simulink model "VDCHyd2020a"  (R2020a)
settings: Solver=daessc  StartTime=0.0  StopTime=simulationEndTime  FixedStep=0.001  RelTol=1e-2
values from neighbouring files (symbols this model uses):
  Bc1_V = [0;0;0;0;0;0]    [initializeSimulationGP.m]
  filtDV = init2ndOrderLowPassFilter(35*2*pi,1,controller.dT)    [initializeLowPassFilters.m]
  filtEnc = init2ndOrderLowPassFilter(35*2*pi,1,controller.dT)    [initializeLowPassFilters.m]
undefined symbols (not defined in the file or in its folder): aux, B11_r_B11Tc1, B11_V, B11_Vr, B11Ftot_r, B12_r_B12Tc2, B12_Rot_Tc2, B12_U_Tc2, B12_V, B12_Vr, B12Ftot_r, B31_r_B31B41, B31_V, B31_Vr, B31FTot_r, B32_r_B32B42, B32_Rot_B42, B32_U_B42, B32_V, B32_Vr, B32FTot_r, B41_r_B41Tc1, B41_V, B41_Vr, B41FTot_r, B42_r_B42Tc2, B42_Rot_Tc2, B42_U_Tc2, B42_V, B42_Vr, B42FTot_r, B52_r_B52P32, B52_Rot_P32, B52_U_P32, B52_V, B52_Vr, B52Ftot_r, Bc1_r_Bc1B11, Bc1_r_Bc1B31, Bc1_Vr, Bc1FTot_r, Bc2_r_Bc2B12, Bc2_r_Bc2B32, Bc2_Rot_B12, Bc2_Rot_B32, Bc2_U_B12, Bc2_U_B32, Bc2_V, Bc2_Vr, Bc2Tot_r, controller, cyl1, cyl2, cylT2, D22_V, D22_Vr, D22Fr, DiscIntNeverNeededParam, dq1, dq11 ... (+125)
libraries: sm_lib x34, nesl_utility x15, simulink x11, dspinverses x1
(part 10 of 12)

== system VDCHyd2020a/sbVDCController/sbFormTotalRequiredForces/sbTotalRequiredForcesRS2/sbFilteredVelocityDerivativeB42/sbDiscreteDerivative3 ==
  u : Inport
  Add : Sum  Inputs=-+
  Gain6 : Gain  Gain=1/(2*controller.dT)
  Integer Delay : Delay  InitialConditionSource=Input port  InitialCondition=0  SampleTime=controller.dT
      settings: InputPortMap=u0,p4
  du/dt : Outport  PortDimensions=1
  wires:
  Add/1 -> Gain6/1
  Integer Delay/1 -> Add/1
  u/1 -> Integer Delay/1, Integer Delay/2, Add/2
  Gain6/1 -> du/dt/1

== system VDCHyd2020a/sbVDCController/sbFormTotalRequiredForces/sbTotalRequiredForcesRS2/sbFilteredVelocityDerivativeB42/sbDiscreteDerivative4 ==
  u : Inport
  Add : Sum  Inputs=-+
  Gain6 : Gain  Gain=1/(2*controller.dT)
  Integer Delay : Delay  InitialConditionSource=Input port  InitialCondition=0  SampleTime=controller.dT
      settings: InputPortMap=u0,p4
  du/dt : Outport  PortDimensions=1
  wires:
  Add/1 -> Gain6/1
  Integer Delay/1 -> Add/1
  u/1 -> Integer Delay/1, Integer Delay/2, Add/2
  Gain6/1 -> du/dt/1

== system VDCHyd2020a/sbVDCController/sbFormTotalRequiredForces/sbTotalRequiredForcesRS2/sbFilteredVelocityDerivativeB42/sbDiscreteDerivative5 ==
  u : Inport
  Add : Sum  Inputs=-+
  Gain6 : Gain  Gain=1/(2*controller.dT)
  Integer Delay : Delay  InitialConditionSource=Input port  InitialCondition=0  SampleTime=controller.dT
      settings: InputPortMap=u0,p4
  du/dt : Outport  PortDimensions=1
  wires:
  Add/1 -> Gain6/1
  Integer Delay/1 -> Add/1
  u/1 -> Integer Delay/1, Integer Delay/2, Add/2
  Gain6/1 -> du/dt/1

== system VDCHyd2020a/sbVDCController/sbFormTotalRequiredForces/sbTotalRequiredForcesRS2/sbFilteredVelocityDerivativeB42/sbDiscreteDerivative6 ==
  u : Inport
  Add : Sum  Inputs=-+
  Gain6 : Gain  Gain=1/(2*controller.dT)
  Integer Delay : Delay  InitialConditionSource=Input port  InitialCondition=0  SampleTime=controller.dT
      settings: InputPortMap=u0,p4
  du/dt : Outport  PortDimensions=1
  wires:
  Add/1 -> Gain6/1
  Integer Delay/1 -> Add/1
  u/1 -> Integer Delay/1, Integer Delay/2, Add/2
  Gain6/1 -> du/dt/1

== system VDCHyd2020a/sbVDCController/sbFormTotalRequiredForces/sbTotalRequiredForcesRS2/sbFilteredVelocityDerivativeB42/sbLowPassFilter1 ==
  dV : Inport
  Delay : Delay  InitialConditionSource=Input port  SampleTime=filtDV.dT
      settings: InputPortMap=u0,p4
  Delay1 : Delay  DelayLength=1  InitialConditionSource=Input port  SampleTime=filtDV.dT
      settings: InputPortMap=u0,p4
  Delay2 : Delay  DelayLength=0  InitialConditionSource=Input port  SampleTime=filtDV.dT
      settings: InputPortMap=u0,p4
  Delay3 : Delay  InitialConditionSource=Input port  SampleTime=filtDV.dT
      settings: InputPortMap=u0,p4
  Delay4 : Delay  DelayLength=1  InitialConditionSource=Input port  SampleTime=filtDV.dT
      settings: InputPortMap=u0,p4
  Gain : Gain  Gain=filtDV.a0
  Gain1 : Gain  Gain=filtDV.b1
  Gain2 : Gain  Gain=filtDV.b2
  Gain3 : Gain  Gain=filtDV.b0
  Gain4 : Gain  Gain=filtDV.a1
  Sum : Sum  Inputs=|--+++
  dVFilt : Outport
  wires:
  Gain3/1 -> Sum/5
  Gain2/1 -> Sum/3
  Delay4/1 -> Gain4/1
  Delay/1 -> Gain/1
  Delay1/1 -> Gain1/1
  Delay2/1 -> Gain2/1
  Gain4/1 -> Sum/1
  Sum/1 -> dVFilt/1, Delay4/1, Delay/1  "dVFilt"
  dV/1 -> Delay2/1, Delay2/2, Delay1/1, Delay3/2, Delay3/1, Delay1/2, Delay4/2, Delay/2  "dV"
  Gain1/1 -> Sum/4
  Gain/1 -> Sum/2
  Delay3/1 -> Gain3/1

== system VDCHyd2020a/sbVDCController/sbFormTotalRequiredForces/sbTotalRequiredForcesRS2/sbFilteredVelocityDerivativeB42/sbLowPassFilter2 ==
  dV : Inport
  Delay : Delay  InitialConditionSource=Input port  SampleTime=filtDV.dT
      settings: InputPortMap=u0,p4
  Delay1 : Delay  DelayLength=1  InitialConditionSource=Input port  SampleTime=filtDV.dT
      settings: InputPortMap=u0,p4
  Delay2 : Delay  DelayLength=0  InitialConditionSource=Input port  SampleTime=filtDV.dT
      settings: InputPortMap=u0,p4
  Delay3 : Delay  InitialConditionSource=Input port  SampleTime=filtDV.dT
      settings: InputPortMap=u0,p4
  Delay4 : Delay  DelayLength=1  InitialConditionSource=Input port  SampleTime=filtDV.dT
      settings: InputPortMap=u0,p4
  Gain : Gain  Gain=filtDV.a0
  Gain1 : Gain  Gain=filtDV.b1
  Gain2 : Gain  Gain=filtDV.b2
  Gain3 : Gain  Gain=filtDV.b0
  Gain4 : Gain  Gain=filtDV.a1
  Sum : Sum  Inputs=|--+++
  dVFilt : Outport
  wires:
  Delay3/1 -> Gain3/1
  Gain/1 -> Sum/2
  Gain1/1 -> Sum/4
  dV/1 -> Delay/2, Delay4/2, Delay1/2, Delay3/1, Delay3/2, Delay1/1, Delay2/2, Delay2/1  "dV"
  Sum/1 -> Delay/1, Delay4/1, dVFilt/1  "dVFilt"
  Gain4/1 -> Sum/1
  Delay2/1 -> Gain2/1
  Delay1/1 -> Gain1/1
  Delay/1 -> Gain/1
  Delay4/1 -> Gain4/1
  Gain2/1 -> Sum/3
  Gain3/1 -> Sum/5

== system VDCHyd2020a/sbVDCController/sbFormTotalRequiredForces/sbTotalRequiredForcesRS2/sbFilteredVelocityDerivativeB42/sbLowPassFilter3 ==
  dV : Inport
  Delay : Delay  InitialConditionSource=Input port  SampleTime=filtDV.dT
      settings: InputPortMap=u0,p4
  Delay1 : Delay  DelayLength=1  InitialConditionSource=Input port  SampleTime=filtDV.dT
      settings: InputPortMap=u0,p4
  Delay2 : Delay  DelayLength=0  InitialConditionSource=Input port  SampleTime=filtDV.dT
      settings: InputPortMap=u0,p4
  Delay3 : Delay  InitialConditionSource=Input port  SampleTime=filtDV.dT
      settings: InputPortMap=u0,p4
  Delay4 : Delay  DelayLength=1  InitialConditionSource=Input port  SampleTime=filtDV.dT
      settings: InputPortMap=u0,p4
  Gain : Gain  Gain=filtDV.a0
  Gain1 : Gain  Gain=filtDV.b1
  Gain2 : Gain  Gain=filtDV.b2
  Gain3 : Gain  Gain=filtDV.b0
  Gain4 : Gain  Gain=filtDV.a1
  Sum : Sum  Inputs=|--+++
  dVFilt : Outport
  wires:
  Gain3/1 -> Sum/5
  Gain2/1 -> Sum/3
  Delay4/1 -> Gain4/1
  Delay/1 -> Gain/1
  Delay1/1 -> Gain1/1
  Delay2/1 -> Gain2/1
  Gain4/1 -> Sum/1
  Sum/1 -> dVFilt/1, Delay4/1, Delay/1  "dVFilt"
  dV/1 -> Delay2/1, Delay2/2, Delay1/1, Delay3/2, Delay3/1, Delay1/2, Delay4/2, Delay/2  "dV"
  Gain1/1 -> Sum/4
  Gain/1 -> Sum/2
  Delay3/1 -> Gain3/1

== system VDCHyd2020a/sbVDCController/sbFormTotalRequiredForces/sbTotalRequiredForcesRS2/sbFilteredVelocityDerivativeB42/sbLowPassFilter4 ==
  dV : Inport
  Delay : Delay  InitialConditionSource=Input port  SampleTime=filtDV.dT
      settings: InputPortMap=u0,p4
  Delay1 : Delay  DelayLength=1  InitialConditionSource=Input port  SampleTime=filtDV.dT
      settings: InputPortMap=u0,p4
  Delay2 : Delay  DelayLength=0  InitialConditionSource=Input port  SampleTime=filtDV.dT
      settings: InputPortMap=u0,p4
  Delay3 : Delay  InitialConditionSource=Input port  SampleTime=filtDV.dT
      settings: InputPortMap=u0,p4
  Delay4 : Delay  DelayLength=1  InitialConditionSource=Input port  SampleTime=filtDV.dT
      settings: InputPortMap=u0,p4
  Gain : Gain  Gain=filtDV.a0
  Gain1 : Gain  Gain=filtDV.b1
  Gain2 : Gain  Gain=filtDV.b2
  Gain3 : Gain  Gain=filtDV.b0
  Gain4 : Gain  Gain=filtDV.a1
  Sum : Sum  Inputs=|--+++
  dVFilt : Outport
  wires:
  Delay3/1 -> Gain3/1
  Gain/1 -> Sum/2
  Gain1/1 -> Sum/4
  dV/1 -> Delay/2, Delay4/2, Delay1/2, Delay3/1, Delay3/2, Delay1/1, Delay2/2, Delay2/1  "dV"
  Sum/1 -> Delay/1, Delay4/1, dVFilt/1  "dVFilt"
  Gain4/1 -> Sum/1
  Delay2/1 -> Gain2/1
  Delay1/1 -> Gain1/1
  Delay/1 -> Gain/1
  Delay4/1 -> Gain4/1
  Gain2/1 -> Sum/3
  Gain3/1 -> Sum/5

== system VDCHyd2020a/sbVDCController/sbFormTotalRequiredForces/sbTotalRequiredForcesRS2/sbFilteredVelocityDerivativeB42/sbLowPassFilter5 ==
  dV : Inport
  Delay : Delay  InitialConditionSource=Input port  SampleTime=filtDV.dT
      settings: InputPortMap=u0,p4
  Delay1 : Delay  DelayLength=1  InitialConditionSource=Input port  SampleTime=filtDV.dT
      settings: InputPortMap=u0,p4
  Delay2 : Delay  DelayLength=0  InitialConditionSource=Input port  SampleTime=filtDV.dT
      settings: InputPortMap=u0,p4
  Delay3 : Delay  InitialConditionSource=Input port  SampleTime=filtDV.dT
      settings: InputPortMap=u0,p4
  Delay4 : Delay  DelayLength=1  InitialConditionSource=Input port  SampleTime=filtDV.dT
      settings: InputPortMap=u0,p4
  Gain : Gain  Gain=filtDV.a0
  Gain1 : Gain  Gain=filtDV.b1
  Gain2 : Gain  Gain=filtDV.b2
  Gain3 : Gain  Gain=filtDV.b0
  Gain4 : Gain  Gain=filtDV.a1
  Sum : Sum  Inputs=|--+++
  dVFilt : Outport
  wires:
  Gain3/1 -> Sum/5
  Gain2/1 -> Sum/3
  Delay4/1 -> Gain4/1
  Delay/1 -> Gain/1
  Delay1/1 -> Gain1/1
  Delay2/1 -> Gain2/1
  Gain4/1 -> Sum/1
  Sum/1 -> dVFilt/1, Delay4/1, Delay/1  "dVFilt"
  dV/1 -> Delay2/1, Delay2/2, Delay1/1, Delay3/2, Delay3/1, Delay1/2, Delay4/2, Delay/2  "dV"
  Gain1/1 -> Sum/4
  Gain/1 -> Sum/2
  Delay3/1 -> Gain3/1

== system VDCHyd2020a/sbVDCController/sbFormTotalRequiredForces/sbTotalRequiredForcesRS2/sbFilteredVelocityDerivativeB42/sbLowPassFilter6 ==
  dV : Inport
  Delay : Delay  InitialConditionSource=Input port  SampleTime=filtDV.dT
      settings: InputPortMap=u0,p4
  Delay1 : Delay  DelayLength=1  InitialConditionSource=Input port  SampleTime=filtDV.dT
      settings: InputPortMap=u0,p4
  Delay2 : Delay  DelayLength=0  InitialConditionSource=Input port  SampleTime=filtDV.dT
      settings: InputPortMap=u0,p4
  Delay3 : Delay  InitialConditionSource=Input port  SampleTime=filtDV.dT
      settings: InputPortMap=u0,p4
  Delay4 : Delay  DelayLength=1  InitialConditionSource=Input port  SampleTime=filtDV.dT
      settings: InputPortMap=u0,p4
  Gain : Gain  Gain=filtDV.a0
  Gain1 : Gain  Gain=filtDV.b1
  Gain2 : Gain  Gain=filtDV.b2
  Gain3 : Gain  Gain=filtDV.b0
  Gain4 : Gain  Gain=filtDV.a1
  Sum : Sum  Inputs=|--+++
  dVFilt : Outport
  wires:
  Delay3/1 -> Gain3/1
  Gain/1 -> Sum/2
  Gain1/1 -> Sum/4
  dV/1 -> Delay/2, Delay4/2, Delay1/2, Delay3/1, Delay3/2, Delay1/1, Delay2/2, Delay2/1  "dV"
  Sum/1 -> Delay/1, Delay4/1, dVFilt/1  "dVFilt"
  Gain4/1 -> Sum/1
  Delay2/1 -> Gain2/1
  Delay1/1 -> Gain1/1
  Delay/1 -> Gain/1
  Delay4/1 -> Gain4/1
  Gain2/1 -> Sum/3
  Gain3/1 -> Sum/5

== system VDCHyd2020a/sbVDCController/sbFormTotalRequiredForces/sbTotalRequiredForcesRS2/sbFilteredVelocityDerivativeBc2/sbDiscreteDerivative1 ==
  u : Inport
  Add : Sum  Inputs=-+
  Gain6 : Gain  Gain=1/(2*controller.dT)
  Integer Delay : Delay  InitialConditionSource=Input port  InitialCondition=0  SampleTime=controller.dT
      settings: InputPortMap=u0,p4
  du/dt : Outport  PortDimensions=1
  wires:
  Add/1 -> Gain6/1
  u/1 -> Integer Delay/1, Integer Delay/2, Add/2
  Integer Delay/1 -> Add/1
  Gain6/1 -> du/dt/1

== system VDCHyd2020a/sbVDCController/sbFormTotalRequiredForces/sbTotalRequiredForcesRS2/sbFilteredVelocityDerivativeBc2/sbDiscreteDerivative2 ==
  u : Inport
  Add : Sum  Inputs=-+
  Gain6 : Gain  Gain=1/(2*controller.dT)
  Integer Delay : Delay  InitialConditionSource=Input port  InitialCondition=0  SampleTime=controller.dT
      settings: InputPortMap=u0,p4
  du/dt : Outport  PortDimensions=1
  wires:
  u/1 -> Integer Delay/1, Integer Delay/2, Add/2
  Integer Delay/1 -> Add/1
  Add/1 -> Gain6/1
  Gain6/1 -> du/dt/1

== system VDCHyd2020a/sbVDCController/sbFormTotalRequiredForces/sbTotalRequiredForcesRS2/sbFilteredVelocityDerivativeBc2/sbDiscreteDerivative3 ==
  u : Inport
  Add : Sum  Inputs=-+
  Gain6 : Gain  Gain=1/(2*controller.dT)
  Integer Delay : Delay  InitialConditionSource=Input port  InitialCondition=0  SampleTime=controller.dT
      settings: InputPortMap=u0,p4
  du/dt : Outport  PortDimensions=1
  wires:
  Add/1 -> Gain6/1
  Integer Delay/1 -> Add/1
  u/1 -> Integer Delay/1, Integer Delay/2, Add/2
  Gain6/1 -> du/dt/1

== system VDCHyd2020a/sbVDCController/sbFormTotalRequiredForces/sbTotalRequiredForcesRS2/sbFilteredVelocityDerivativeBc2/sbDiscreteDerivative4 ==
  u : Inport
  Add : Sum  Inputs=-+
  Gain6 : Gain  Gain=1/(2*controller.dT)
  Integer Delay : Delay  InitialConditionSource=Input port  InitialCondition=0  SampleTime=controller.dT
      settings: InputPortMap=u0,p4
  du/dt : Outport  PortDimensions=1
  wires:
  Add/1 -> Gain6/1
  Integer Delay/1 -> Add/1
  u/1 -> Integer Delay/1, Integer Delay/2, Add/2
  Gain6/1 -> du/dt/1

== system VDCHyd2020a/sbVDCController/sbFormTotalRequiredForces/sbTotalRequiredForcesRS2/sbFilteredVelocityDerivativeBc2/sbDiscreteDerivative5 ==
  u : Inport
  Add : Sum  Inputs=-+
  Gain6 : Gain  Gain=1/(2*controller.dT)
  Integer Delay : Delay  InitialConditionSource=Input port  InitialCondition=0  SampleTime=controller.dT
      settings: InputPortMap=u0,p4
  du/dt : Outport  PortDimensions=1
  wires:
  Add/1 -> Gain6/1
  Integer Delay/1 -> Add/1
  u/1 -> Integer Delay/1, Integer Delay/2, Add/2
  Gain6/1 -> du/dt/1

== system VDCHyd2020a/sbVDCController/sbFormTotalRequiredForces/sbTotalRequiredForcesRS2/sbFilteredVelocityDerivativeBc2/sbDiscreteDerivative6 ==
  u : Inport
  Add : Sum  Inputs=-+
  Gain6 : Gain  Gain=1/(2*controller.dT)
  Integer Delay : Delay  InitialConditionSource=Input port  InitialCondition=0  SampleTime=controller.dT
      settings: InputPortMap=u0,p4
  du/dt : Outport  PortDimensions=1
  wires:
  Add/1 -> Gain6/1
  Integer Delay/1 -> Add/1
  u/1 -> Integer Delay/1, Integer Delay/2, Add/2
  Gain6/1 -> du/dt/1

== system VDCHyd2020a/sbVDCController/sbFormTotalRequiredForces/sbTotalRequiredForcesRS2/sbFilteredVelocityDerivativeBc2/sbLowPassFilter1 ==
  dV : Inport
  Delay : Delay  InitialConditionSource=Input port  SampleTime=filtDV.dT
      settings: InputPortMap=u0,p4
  Delay1 : Delay  DelayLength=1  InitialConditionSource=Input port  SampleTime=filtDV.dT
      settings: InputPortMap=u0,p4
  Delay2 : Delay  DelayLength=0  InitialConditionSource=Input port  SampleTime=filtDV.dT
      settings: InputPortMap=u0,p4
  Delay3 : Delay  InitialConditionSource=Input port  SampleTime=filtDV.dT
      settings: InputPortMap=u0,p4
  Delay4 : Delay  DelayLength=1  InitialConditionSource=Input port  SampleTime=filtDV.dT
      settings: InputPortMap=u0,p4
  Gain : Gain  Gain=filtDV.a0
  Gain1 : Gain  Gain=filtDV.b1
  Gain2 : Gain  Gain=filtDV.b2
  Gain3 : Gain  Gain=filtDV.b0
  Gain4 : Gain  Gain=filtDV.a1
  Sum : Sum  Inputs=|--+++
  dVFilt : Outport
  wires:
  Gain3/1 -> Sum/5
  Gain2/1 -> Sum/3
  Delay4/1 -> Gain4/1
  Delay/1 -> Gain/1
  Delay1/1 -> Gain1/1
  Delay2/1 -> Gain2/1
  Gain4/1 -> Sum/1
  Sum/1 -> dVFilt/1, Delay4/1, Delay/1  "dVFilt"
  dV/1 -> Delay2/1, Delay2/2, Delay1/1, Delay3/2, Delay3/1, Delay1/2, Delay4/2, Delay/2  "dV"
  Gain1/1 -> Sum/4
  Gain/1 -> Sum/2
  Delay3/1 -> Gain3/1

== system VDCHyd2020a/sbVDCController/sbFormTotalRequiredForces/sbTotalRequiredForcesRS2/sbFilteredVelocityDerivativeBc2/sbLowPassFilter2 ==
  dV : Inport
  Delay : Delay  InitialConditionSource=Input port  SampleTime=filtDV.dT
      settings: InputPortMap=u0,p4
  Delay1 : Delay  DelayLength=1  InitialConditionSource=Input port  SampleTime=filtDV.dT
      settings: InputPortMap=u0,p4
  Delay2 : Delay  DelayLength=0  InitialConditionSource=Input port  SampleTime=filtDV.dT
      settings: InputPortMap=u0,p4
  Delay3 : Delay  InitialConditionSource=Input port  SampleTime=filtDV.dT
      settings: InputPortMap=u0,p4
  Delay4 : Delay  DelayLength=1  InitialConditionSource=Input port  SampleTime=filtDV.dT
      settings: InputPortMap=u0,p4
  Gain : Gain  Gain=filtDV.a0
  Gain1 : Gain  Gain=filtDV.b1
  Gain2 : Gain  Gain=filtDV.b2
  Gain3 : Gain  Gain=filtDV.b0
  Gain4 : Gain  Gain=filtDV.a1
  Sum : Sum  Inputs=|--+++
  dVFilt : Outport
  wires:
  Delay3/1 -> Gain3/1
  Gain/1 -> Sum/2
  Gain1/1 -> Sum/4
  dV/1 -> Delay/2, Delay4/2, Delay1/2, Delay3/1, Delay3/2, Delay1/1, Delay2/2, Delay2/1  "dV"
  Sum/1 -> Delay/1, Delay4/1, dVFilt/1  "dVFilt"
  Gain4/1 -> Sum/1
  Delay2/1 -> Gain2/1
  Delay1/1 -> Gain1/1
  Delay/1 -> Gain/1
  Delay4/1 -> Gain4/1
  Gain2/1 -> Sum/3
  Gain3/1 -> Sum/5

== system VDCHyd2020a/sbVDCController/sbFormTotalRequiredForces/sbTotalRequiredForcesRS2/sbFilteredVelocityDerivativeBc2/sbLowPassFilter3 ==
  dV : Inport
  Delay : Delay  InitialConditionSource=Input port  SampleTime=filtDV.dT
      settings: InputPortMap=u0,p4
  Delay1 : Delay  DelayLength=1  InitialConditionSource=Input port  SampleTime=filtDV.dT
      settings: InputPortMap=u0,p4
  Delay2 : Delay  DelayLength=0  InitialConditionSource=Input port  SampleTime=filtDV.dT
      settings: InputPortMap=u0,p4
  Delay3 : Delay  InitialConditionSource=Input port  SampleTime=filtDV.dT
      settings: InputPortMap=u0,p4
  Delay4 : Delay  DelayLength=1  InitialConditionSource=Input port  SampleTime=filtDV.dT
      settings: InputPortMap=u0,p4
  Gain : Gain  Gain=filtDV.a0
  Gain1 : Gain  Gain=filtDV.b1
  Gain2 : Gain  Gain=filtDV.b2
  Gain3 : Gain  Gain=filtDV.b0
  Gain4 : Gain  Gain=filtDV.a1
  Sum : Sum  Inputs=|--+++
  dVFilt : Outport
  wires:
  Gain3/1 -> Sum/5
  Gain2/1 -> Sum/3
  Delay4/1 -> Gain4/1
  Delay/1 -> Gain/1
  Delay1/1 -> Gain1/1
  Delay2/1 -> Gain2/1
  Gain4/1 -> Sum/1
  Sum/1 -> dVFilt/1, Delay4/1, Delay/1  "dVFilt"
  dV/1 -> Delay2/1, Delay2/2, Delay1/1, Delay3/2, Delay3/1, Delay1/2, Delay4/2, Delay/2  "dV"
  Gain1/1 -> Sum/4
  Gain/1 -> Sum/2
  Delay3/1 -> Gain3/1

== system VDCHyd2020a/sbVDCController/sbFormTotalRequiredForces/sbTotalRequiredForcesRS2/sbFilteredVelocityDerivativeBc2/sbLowPassFilter4 ==
  dV : Inport
  Delay : Delay  InitialConditionSource=Input port  SampleTime=filtDV.dT
      settings: InputPortMap=u0,p4
  Delay1 : Delay  DelayLength=1  InitialConditionSource=Input port  SampleTime=filtDV.dT
      settings: InputPortMap=u0,p4
  Delay2 : Delay  DelayLength=0  InitialConditionSource=Input port  SampleTime=filtDV.dT
      settings: InputPortMap=u0,p4
  Delay3 : Delay  InitialConditionSource=Input port  SampleTime=filtDV.dT
      settings: InputPortMap=u0,p4
  Delay4 : Delay  DelayLength=1  InitialConditionSource=Input port  SampleTime=filtDV.dT
      settings: InputPortMap=u0,p4
  Gain : Gain  Gain=filtDV.a0
  Gain1 : Gain  Gain=filtDV.b1
  Gain2 : Gain  Gain=filtDV.b2
  Gain3 : Gain  Gain=filtDV.b0
  Gain4 : Gain  Gain=filtDV.a1
  Sum : Sum  Inputs=|--+++
  dVFilt : Outport
  wires:
  Delay3/1 -> Gain3/1
  Gain/1 -> Sum/2
  Gain1/1 -> Sum/4
  dV/1 -> Delay/2, Delay4/2, Delay1/2, Delay3/1, Delay3/2, Delay1/1, Delay2/2, Delay2/1  "dV"
  Sum/1 -> Delay/1, Delay4/1, dVFilt/1  "dVFilt"
  Gain4/1 -> Sum/1
  Delay2/1 -> Gain2/1
  Delay1/1 -> Gain1/1
  Delay/1 -> Gain/1
  Delay4/1 -> Gain4/1
  Gain2/1 -> Sum/3
  Gain3/1 -> Sum/5

== system VDCHyd2020a/sbVDCController/sbFormTotalRequiredForces/sbTotalRequiredForcesRS2/sbFilteredVelocityDerivativeBc2/sbLowPassFilter5 ==
  dV : Inport
  Delay : Delay  InitialConditionSource=Input port  SampleTime=filtDV.dT
      settings: InputPortMap=u0,p4
  Delay1 : Delay  DelayLength=1  InitialConditionSource=Input port  SampleTime=filtDV.dT
      settings: InputPortMap=u0,p4
  Delay2 : Delay  DelayLength=0  InitialConditionSource=Input port  SampleTime=filtDV.dT
      settings: InputPortMap=u0,p4
  Delay3 : Delay  InitialConditionSource=Input port  SampleTime=filtDV.dT
      settings: InputPortMap=u0,p4
  Delay4 : Delay  DelayLength=1  InitialConditionSource=Input port  SampleTime=filtDV.dT
      settings: InputPortMap=u0,p4
  Gain : Gain  Gain=filtDV.a0
  Gain1 : Gain  Gain=filtDV.b1
  Gain2 : Gain  Gain=filtDV.b2
  Gain3 : Gain  Gain=filtDV.b0
  Gain4 : Gain  Gain=filtDV.a1
  Sum : Sum  Inputs=|--+++
  dVFilt : Outport
  wires:
  Gain3/1 -> Sum/5
  Gain2/1 -> Sum/3
  Delay4/1 -> Gain4/1
  Delay/1 -> Gain/1
  Delay1/1 -> Gain1/1
  Delay2/1 -> Gain2/1
  Gain4/1 -> Sum/1
  Sum/1 -> dVFilt/1, Delay4/1, Delay/1  "dVFilt"
  dV/1 -> Delay2/1, Delay2/2, Delay1/1, Delay3/2, Delay3/1, Delay1/2, Delay4/2, Delay/2  "dV"
  Gain1/1 -> Sum/4
  Gain/1 -> Sum/2
  Delay3/1 -> Gain3/1

== system VDCHyd2020a/sbVDCController/sbFormTotalRequiredForces/sbTotalRequiredForcesRS2/sbFilteredVelocityDerivativeBc2/sbLowPassFilter6 ==
  dV : Inport
  Delay : Delay  InitialConditionSource=Input port  SampleTime=filtDV.dT
      settings: InputPortMap=u0,p4
  Delay1 : Delay  DelayLength=1  InitialConditionSource=Input port  SampleTime=filtDV.dT
      settings: InputPortMap=u0,p4
  Delay2 : Delay  DelayLength=0  InitialConditionSource=Input port  SampleTime=filtDV.dT
      settings: InputPortMap=u0,p4
  Delay3 : Delay  InitialConditionSource=Input port  SampleTime=filtDV.dT
      settings: InputPortMap=u0,p4
  Delay4 : Delay  DelayLength=1  InitialConditionSource=Input port  SampleTime=filtDV.dT
      settings: InputPortMap=u0,p4
  Gain : Gain  Gain=filtDV.a0
  Gain1 : Gain  Gain=filtDV.b1
  Gain2 : Gain  Gain=filtDV.b2
  Gain3 : Gain  Gain=filtDV.b0
  Gain4 : Gain  Gain=filtDV.a1
  Sum : Sum  Inputs=|--+++
  dVFilt : Outport
  wires:
  Delay3/1 -> Gain3/1
  Gain/1 -> Sum/2
  Gain1/1 -> Sum/4
  dV/1 -> Delay/2, Delay4/2, Delay1/2, Delay3/1, Delay3/2, Delay1/1, Delay2/2, Delay2/1  "dV"
  Sum/1 -> Delay/1, Delay4/1, dVFilt/1  "dVFilt"
  Gain4/1 -> Sum/1
  Delay2/1 -> Gain2/1
  Delay1/1 -> Gain1/1
  Delay/1 -> Gain/1
  Delay4/1 -> Gain4/1
  Gain2/1 -> Sum/3
  Gain3/1 -> Sum/5

== system VDCHyd2020a/sbVDCController/sbFormAnalyticQuantities/sbRevoluteSegment1/sbGeomPropRS1/sbq1AngleRate/sbDiscreteDerivative ==
  note: Overview of different differentiation scheme can be found in:
      | Harrison, A. J. L., and D. P. Stoten. "Generalized finite difference methods for optimal estimation of derivatives in real-time control problems." Proceedings of the institution of mechanical engineers, part I: journal of systems and control engineering 209.2 (1995): 67-78.
  q1Angle : Inport
  Add : Sum  Inputs=-+
  Gain6 : Gain  Gain=1/(2*controller.dT)
  Integer Delay : Delay  InitialConditionSource=Input port  InitialCondition=0  SampleTime=controller.dT
      settings: InputPortMap=u0,p4
  q1AngleRate : Outport  PortDimensions=1
  wires:
  q1Angle/1 -> Integer Delay/1, Integer Delay/2, Add/2
  Gain6/1 -> q1AngleRate/1
  Integer Delay/1 -> Add/1
  Add/1 -> Gain6/1

== system VDCHyd2020a/sbVDCController/sbFormAnalyticQuantities/sbRevoluteSegment2/sbGeomPropRS2/sbq2AngleRate/sbDiscreteDerivative ==
  q2Angle : Inport
  Add : Sum  Inputs=-+
  Gain6 : Gain  Gain=1/(2*controller.dT)
  Integer Delay : Delay  InitialConditionSource=Input port  InitialCondition=0  SampleTime=controller.dT
      settings: InputPortMap=u0,p4
  q2AngleRate : Outport  PortDimensions=1
  wires:
  q2Angle/1 -> Integer Delay/1, Integer Delay/2, Add/2
  Gain6/1 -> q2AngleRate/1
  Integer Delay/1 -> Add/1
  Add/1 -> Gain6/1

== matlab function VDCHyd2020a/sbVDCController/sbFormAnalyticQuantities/sbRevoluteSegment1/sbGeomPropRS1/sbLiftPistonStroke/liftPistonStroke ==
  data: q1 input; x1 output; geom parameter; cyl1 parameter
function x1 = liftPistonStroke(q1, geom, cyl1)

    % Calculates lift piston stroke per the paper equation (18).
    x1 = sqrt(geom.L1*geom.L1+geom.L11*geom.L11+2*geom.L1*geom.L11*cos(q1))-cyl1.x0;

end

== matlab function VDCHyd2020a/sbVDCController/sbFormAnalyticQuantities/sbRevoluteSegment1/sbGeomPropRS1/sbq11AngleValue/q11AngleValue ==
  data: x1 input; q11 output; geom parameter; cyl1 parameter
function q11 = q11AngleValue(x1, geom, cyl1)

    % Calculates q11-angle per the paper equation (19).
    q11 = -acos((geom.L11*geom.L11-(x1+cyl1.x0)*(x1+cyl1.x0)-geom.L1*geom.L1)/(-2*(x1+cyl1.x0)*geom.L1));

end

== matlab function VDCHyd2020a/sbVDCController/sbAuxiliaryJointAngles/q1Angle ==
  data: theta1 input; q1 output; geom parameter
function q1 = q1Angle(theta1, geom)

    % Calculates q1 angle value from the encoder- (or other by means-)
    % obtained angle theta1. 
    q1 = -pi/2 - geom.beta1 - geom.beta2 + theta1;

end

== matlab function VDCHyd2020a/sbVDCController/sbAuxiliaryJointAngles/q2Angle ==
  data: theta2 input; q2 output; geom parameter
function q2 = q2Angle(theta2, geom)

    % Calculates q2 angle value from the encoder- (or other by means-)
    % obtained angle Theta2.
    q2 = theta2 - geom.beta3 - geom.beta4;

end

== matlab function VDCHyd2020a/sbHydraulicElements/sbValveFlowsPS1/extensionValveFlows ==
  data: pat2 input; Qat2 output; pbt2 input; ut2v input; pS input; pR input; Qbt2 output; valveT2 parameter
function [Qat2, Qbt2] = extensionValveFlows(pat2, pbt2, ut2v, pS, pR, valveT2)

    % Calculates extension valve flows per the paper equations (82) and (83).
    Qat2 = valveT2.cp1*sqAbsPresDrop(pS - pat2)*ut2v*selFcn(ut2v) + ...
       valveT2.cn1*sqAbsPresDrop(pat2 - pR)*ut2v*selFcn(-ut2v);
    Qbt2 = -valveT2.cn2*sqAbsPresDrop(pbt2 - pR)*ut2v*selFcn(ut2v) - ...
       valveT2.cp2*sqAbsPresDrop(pS - pbt2)*ut2v*selFcn(-ut2v);
   
end

function S = selFcn(U)

    % Implements the selection function (84). 
    if U > 0
        S = 1;
    else
        S = 0;
    end
    
end

function nup = sqAbsPresDrop(dp)

    % Implements the pressure drop function (85).
    nup = sign(dp)*sqrt(abs(dp));

end

== matlab function VDCHyd2020a/sbVDCController/sbFormAnalyticQuantities/sbRevoluteSegment1/sbGeomPropRS1/sbq12AngleValue/q12AngleValue ==
  data: x1 input; q12 output; geom parameter; cyl1 parameter
function q12 = q12AngleValue(x1, geom, cyl1)

    % Calculates q12-angle per the paper equation (20).
    q12 = -acos((geom.L1*geom.L1-(x1+cyl1.x0)*(x1+cyl1.x0)-geom.L11*geom.L11)/(-2*(x1+cyl1.x0)*geom.L11));

end

== matlab function VDCHyd2020a/sbVDCController/sbFormAnalyticQuantities/sbRevoluteSegment2/sbGeomPropRS2/sbq21AngleValue/q21AngleValue ==
  data: x2 input; q21 output; geom parameter; cyl2 parameter
function q21 = q21AngleValue(x2, geom, cyl2)

    % Calculates q21-angle per the paper equation (19).
    q21 = -acos((geom.L21*geom.L21-(x2+cyl2.x0)*(x2+cyl2.x0)-geom.L2*geom.L2)/(-2*(x2+cyl2.x0)*geom.L2));

end

== matlab function VDCHyd2020a/sbVDCController/sbFormAnalyticQuantities/sbRevoluteSegment2/sbGeomPropRS2/sbq21AngleRate/q21AngleRate ==
  data: x2 input; q21 input; dx2 input; dq21 output; geom parameter; cyl2 parameter
function dq21 = q21AngleRate(x2, q21, dx2, geom, cyl2)
    
    % Calculates q21 angle rate per the paper equation (22).
    dq21 = -((x2+cyl2.x0)-geom.L2*cos(q21))/((x2+cyl2.x0)*geom.L2*sin(q21))*dx2;

end

== matlab function VDCHyd2020a/sbVDCController/sbFormAnalyticQuantities/sbRevoluteSegment2/sbGeomPropRS2/sbTiltPistonVelocity/tiltPistonVelocity ==
  data: dq2 input; x2 input; q2 input; dx2 output; geom parameter; cyl2 parameter
function dx2 = tiltPistonVelocity(dq2, x2, q2, geom, cyl2)

    % Calculates lift piston velocity per the paper equation (21).
    dx2 = -(geom.L2*geom.L21*sin(q2))/(x2+cyl2.x0)*dq2;

end

== matlab function VDCHyd2020a/sbVDCController/sbFormAnalyticQuantities/sbRevoluteSegment2/sbGeomPropRS2/sbq22AngleValue/q22AngleValue ==
  data: x2 input; q22 output; geom parameter; cyl2 parameter
function q22 = q22AngleValue(x2, geom, cyl2)

    % Calculates q22-angle per the paper equation (20).
    q22 = -acos((geom.L2*geom.L2-(x2+cyl2.x0)*(x2+cyl2.x0)-geom.L21*geom.L21)/(-2*(x2+cyl2.x0)*geom.L21));

end

== matlab function VDCHyd2020a/sbVDCController/sbFormAnalyticQuantities/sbRevoluteSegment2/sbGeomPropRS2req/sbRequiredq21AngleRate/requiredq21AngleRate ==
  data: x2 input; q21 input; dx2r input; dq21r output; geom parameter; cyl2 parameter
function dq21r = requiredq21AngleRate(x2, q21, dx2r, geom, cyl2)

    % Calculate the required q21 angle rate per the paper equation (22).
    dq21r = -((x2+cyl2.x0)-geom.L2*cos(q21))/((x2+cyl2.x0)*geom.L2*sin(q21))*dx2r;

end

== matlab function VDCHyd2020a/sbVDCController/sbFormAnalyticQuantities/sbRevoluteSegment2/sbGeomPropRS2/sbq22AngleRate/q22AngleRate ==
  data: x2 input; q22 input; dx2 input; dq22 output; geom parameter; cyl2 parameter
function dq22 = q22AngleRate(x2, q22, dx2, geom, cyl2)

    % Calculates q22 angle rate per the paper equation (23). 
    dq22 = -((x2+cyl2.x0)-geom.L21*cos(q22))/((x2+cyl2.x0)*geom.L21*sin(q22))*dx2;

end

== matlab function VDCHyd2020a/sbVDCController/sbFormAnalyticQuantities/sbRevoluteSegment2/sbGeomPropRS2req/sbRequiredq22AngleRate/requiredq22AngleRate ==
  data: x2 input; q22 input; dx2r input; dq22r output; geom parameter; cyl2 parameter
function dq22r = requiredq22AngleRate(x2, q22, dx2r, geom, cyl2)

    % Calculates the required q12 angle rate per the paper equation (23).
    dq22r = -((x2+cyl2.x0)-geom.L21*cos(q22))/((x2+cyl2.x0)*geom.L21*sin(q22))*dx2r;

end

== matlab function VDCHyd2020a/sbVDCController/sbFormAnalyticQuantities/sbRevoluteSegment2/sbGeomPropRS2/sbTiltPistonStroke/tiltPistonStroke ==
  data: q2 input; x2 output; geom parameter; cyl2 parameter
function x2 = tiltPistonStroke(q2, geom, cyl2)

    % Calculates lift piston stroke per the paper equation (18).
    x2 = sqrt(geom.L2*geom.L2+geom.L21*geom.L21+2*geom.L2*geom.L21*cos(q2))-cyl2.x0;

end

== matlab function VDCHyd2020a/sbHydraulicManipulatorSimscape/sbLiftCylinderAndLiftPiston/sbFrictionForceRS1/sbFrictionRegressorRS1/frictionRegressorFunctionRS1 ==
  data: v input; z input; Yf output; L input; Fd input; frictionRS1 parameter
function Yf = frictionRegressor(v,z,L, Fd, frictionRS1)

    % Forms the friction regressor from Zhu, W. H., & Piedboeuf, J. C. 
    % (2005). Adaptive output force tracking control of hydraulic cylinders 
    % with applications to robot manipulators.
    Yf = [(1 - L)*g(z, frictionRS1.zss)*S(z),...
          -(1 - L)*g(-z, frictionRS1.zss)*S(-z),...
          1 - L,...
          (1 - L)*S(v)*phivp(v)*v,...
          (1 - L)*S(-v)*phivn(v)*v,...
          S(Fd)*L*phifp(Fd,frictionRS1.deltap),...
          S(-Fd)*L*phifn(Fd,frictionRS1.deltan)];

end

function S = S(x)

    % Per (2) from Zhu, W. H., & Piedboeuf, J. C. (2005).
    if x > 0
        S = 1;
    else
        S = 0;
    end

end

function g = g(z, zss)

    % Per (5) in Zhu, W. H., & Piedboeuf, J. C. (2005).
    if z >= zss
        g = 1;
    elseif z <= 0
        g = 0;
    else
        g = z/zss;
    end

end

function phifp = phifp(f, deltafp)

    % Per (6) in Zhu, W. H., & Piedboeuf, J. C. (2005).
    phifp = f/(1 + deltafp*abs(f));

end

function phifn = phifn(f, deltafn)

    % Per (6) in Zhu, W. H., & Piedboeuf, J. C. (2005).
    phifn = f/(1 + deltafn*abs(f));

end

function phivp = phivp(v)

    % Chosen as constant. More details on pp. 211 of Zhu, W. H., & 
    % Piedboeuf, J. C. (2005), just above Eq. (71)
    phivp = 5 + 0*v;

end

function phivn = phivn(v)

    % Chosen as constant. More details on pp. 211 of Zhu, W. H., & 
    % Piedboeuf, J. C. (2005), just above Eq. (71)
    phivn = 5 + 0*v;

end

== matlab function VDCHyd2020a/sbVDCController/sbFormAnalyticQuantities/sbRevoluteSegment2/sbGeomPropRS2req/sbRequiredTiltPistonVelocity/requiredTiltPistonVelocity ==
  data: dq2r input; x2 input; q2 input; dx2r output; geom parameter; cyl2 parameter
function dx2r = requiredTiltPistonVelocity(dq2r, x2, q2, geom, cyl2)

    % calculates required lift piston velocity per the paper equation (21).
    dx2r = -(geom.L2*geom.L21*sin(q2))/(x2+cyl2.x0)*dq2r;

end

== matlab function VDCHyd2020a/sbHydraulicManipulatorSimscape/sbTiltCylinderAndTiltPiston/sbFrictionForceRS2/sbFrictionRegressorRS2/frictionRegressorFunctionRS2 ==
  data: v input; z input; Yf output; L input; Fd input; frictionRS2 parameter
function Yf = frictionRegressor(v,z,L, Fd, frictionRS2)

    % Forms the friction regressor from Zhu, W. H., & Piedboeuf, J. C. 
    % (2005). Adaptive output force tracking control of hydraulic cylinders 
    % with applications to robot manipulators.
    Yf = [(1 - L)*g(z, frictionRS2.zss)*S(z),...
          -(1 - L)*g(-z, frictionRS2.zss)*S(-z),...
          1 - L,...
          (1 - L)*S(v)*phivp(v)*v,...
          (1 - L)*S(-v)*phivn(v)*v,...
          S(Fd)*L*phifp(Fd,frictionRS2.deltap),...
          S(-Fd)*L*phifn(Fd,frictionRS2.deltan)];

end

function S = S(x)

    % Per (2) from Zhu, W. H., & Piedboeuf, J. C. (2005).
    if x > 0
        S = 1;
    else
        S = 0;
    end

end

function g = g(z, zss)

    % Per (5) in Zhu, W. H., & Piedboeuf, J. C. (2005).
    if z >= zss
        g = 1;
    elseif z <= 0
        g = 0;
    else
        g = z/zss;
    end

end

function phifp = phifp(f, deltafp)

    % Per (6) in Zhu, W. H., & Piedboeuf, J. C. (2005).
    phifp = f/(1 + deltafp*abs(f));

end

function phifn = phifn(f, deltafn)

    % Per (6) in Zhu, W. H., & Piedboeuf, J. C. (2005).
    phifn = f/(1 + deltafn*abs(f));

end

function phivp = phivp(v)

    % Chosen as constant. More details on pp. 211 of Zhu, W. H., & 
    % Piedboeuf, J. C. (2005), just above Eq. (71)
    phivp = 5 + 0*v;

end

function phivn = phivn(v)

    % Chosen as constant. More details on pp. 211 of Zhu, W. H., & 
    % Piedboeuf, J. C. (2005), just above Eq. (71)
    phivn = 5 + 0*v;

end

== matlab function VDCHyd2020a/sbVDCController/sbFormingControlActions/controlVoltageRS2 ==
  data: uf2r input; pS input; pR input; pa2 input; pb2 input; x2 input; u2 output; thetav2 input; hosing2 parameter; cyl2 parameter
function u2  = calculateControlVoltage(uf2r, pS, pR, pa2, pb2, x2, thetav2, hosing2, cyl2)

    cp1 = thetav2(1); cn1 = thetav2(2); cp2 = thetav2(3); cn2 = thetav2(4);

    % Implemented per (27) in S. Lampinen, J. Koivumäki and J. Mattila, 
    % "Improved Hydraulic Cylinder Model for the Virtual Decomposition 
    % Control Approach," 2019 IEEE International Conference on Cybernetics 
    % and Intelligent Systems (CIS) and IEEE Conference on Robotics, 
    % Automation and Mechatronics (RAM), Bangkok, Thailand, 2019, 
    % pp. 113-118, doi: 10.1109/CIS-RAM47153.2019.9095788 
    u2 = uf2r*selFcn(uf2r)/( (cp1*sqAbsPresDrop(pS-pa2))/(hosing2.V0a/cyl2.Aa + x2) + (cn2*sqAbsPresDrop(pb2-pR))/(hosing2.V0b/cyl2.Ab + cyl2.sp - x2) ) + ...
         uf2r*selFcn(-uf2r)/( (cp2*sqAbsPresDrop(pS-pb2))/(hosing2.V0b/cyl2.Ab + cyl2.sp - x2) + (cn1*sqAbsPresDrop(pa2-pR))/(hosing2.V0a/cyl2.Aa + x2) );


end


function S = selFcn(U)

    if U > 0
        S = 1;
    else
        S = 0;
    end
    
end

function nup = sqAbsPresDrop(dp)

    nup = sign(dp)*sqrt(abs(dp));

end

== matlab function VDCHyd2020a/sbHydraulicManipulatorSimscape/sbPrismaticJointCylinderAndPiston/sbFrictionForcePS2/sbFrictionRegressorPS2/frictionRegressorFunctionPS2 ==
  data: v input; z input; Yf output; L input; Fd input; frictionPS2 parameter
function Yf = frictionRegressor(v,z,L, Fd, frictionPS2)

    % Forms the friction regressor from Zhu, W. H., & Piedboeuf, J. C. 
    % (2005). Adaptive output force tracking control of hydraulic cylinders 
    % with applications to robot manipulators.
    Yf = [(1 - L)*g(z, frictionPS2.zss)*S(z),...
          -(1 - L)*g(-z, frictionPS2.zss)*S(-z),...
          1 - L,...
          (1 - L)*S(v)*phivp(v)*v,...
          (1 - L)*S(-v)*phivn(v)*v,...
          S(Fd)*L*phifp(Fd,frictionPS2.deltap),...
          S(-Fd)*L*phifn(Fd,frictionPS2.deltan)];

end

function S = S(x)

    % Per (2) from Zhu, W. H., & Piedboeuf, J. C. (2005).
    if x > 0
        S = 1;
    else
        S = 0;
    end

end

function g = g(z, zss)

    % Per (5) in Zhu, W. H., & Piedboeuf, J. C. (2005).
    if z >= zss
        g = 1;
    elseif z <= 0
        g = 0;
    else
        g = z/zss;
    end

end

function phifp = phifp(f, deltafp)

    % Per (6) in Zhu, W. H., & Piedboeuf, J. C. (2005).
    phifp = f/(1 + deltafp*abs(f));

end

function phifn = phifn(f, deltafn)

    % Per (6) in Zhu, W. H., & Piedboeuf, J. C. (2005).
    phifn = f/(1 + deltafn*abs(f));

end

function phivp = phivp(v)

    % Chosen as constant. More details on pp. 211 of Zhu, W. H., & 
    % Piedboeuf, J. C. (2005), just above Eq. (71)
    phivp = 5 + 0*v;

end

function phivn = phivn(v)

    % Chosen as constant. More details on pp. 211 of Zhu, W. H., & 
    % Piedboeuf, J. C. (2005), just above Eq. (71)
    phivn = 5 + 0*v;

end

== matlab function VDCHyd2020a/sbCartesianControl/velocityJacobianFunction ==
  data: theta1 input; J output; theta2 input; xt2 input
function J = velocityJacobian(theta1, theta2, xt2)

    % Velocity Jacobian matrix in the present example, relating the TCP
    % velocity in the world frame with joint velocities.
    % W_V_D22 = J * q'
    % The derivation is provided in the supplementary pdf.
    J11 = -0.1*cos(theta1) - 0.152638*cos(theta1+theta2) - 1.59687*sin(theta1) + (-1.99949 - xt2)*sin(theta1 + theta2);
    J12 = -0.152638*cos(theta1 + theta2) + (-1.99949 - xt2)*sin(theta1 + theta2);
    J13 = cos(theta1 + theta2);
    J21 = cos(theta1)*(1.59687 + (1.99949 + xt2) * cos(theta2) - 0.154167*sin(theta2)) + sin(theta1)*(-0.1 - 0.154167*cos(theta2) + (-1.99949-xt2)*sin(theta2));
    J22 = cos(theta1)*((1.99949 + xt2)*cos(theta2) - 0.154167*sin(theta2)) + sin(theta1)*(-0.154167*cos(theta2) + (-1.99949 - xt2)*sin(theta2));
    J23 = cos(theta2)*sin(theta1) + cos(theta1)*sin(theta2);
    J = [J11 J12 J13; J21 J22 J23];

end

== matlab function VDCHyd2020a/sbVDCController/sbFormingControlActions/sbFrictionRegressorPS2/frictionRegressorFunctionPS2 ==
  data: v input; z input; Yf output; L input; Fd input; frictionPS2 parameter
function Yf = frictionRegressor(v,z,L, Fd, frictionPS2)

    % Forms the friction regressor from Zhu, W. H., & Piedboeuf, J. C. 
    % (2005). Adaptive output force tracking control of hydraulic cylinders 
    % with applications to robot manipulators.
    Yf = [(1 - L)*g(z, frictionPS2.zss)*S(z),...
          -(1 - L)*g(-z, frictionPS2.zss)*S(-z),...
          1 - L,...
          (1 - L)*S(v)*phivp(v)*v,...
          (1 - L)*S(-v)*phivn(v)*v,...
          S(Fd)*L*phifp(Fd,frictionPS2.deltap),...
          S(-Fd)*L*phifn(Fd,frictionPS2.deltan)];

end

function S = S(x)

    % Per (2) from Zhu, W. H., & Piedboeuf, J. C. (2005).
    if x > 0
        S = 1;
    else
        S = 0;
    end

end

function g = g(z, zss)

    % Per (5) in Zhu, W. H., & Piedboeuf, J. C. (2005).
    if z >= zss
        g = 1;
    elseif z <= 0
        g = 0;
    else
        g = z/zss;
    end

end

function phifp = phifp(f, deltafp)

    % Per (6) in Zhu, W. H., & Piedboeuf, J. C. (2005).
    phifp = f/(1 + deltafp*abs(f));

end

function phifn = phifn(f, deltafn)

    % Per (6) in Zhu, W. H., & Piedboeuf, J. C. (2005).
    phifn = f/(1 + deltafn*abs(f));

end

function phivp = phivp(v)

    % Chosen as constant. More details on pp. 211 of Zhu, W. H., & 
    % Piedboeuf, J. C. (2005), just above Eq. (71)
    phivp = 5 + 0*v;

end

function phivn = phivn(v)

    % Chosen as constant. More details on pp. 211 of Zhu, W. H., & 
    % Piedboeuf, J. C. (2005), just above Eq. (71)
    phivn = 5 + 0*v;

end

== matlab function VDCHyd2020a/sbVDCController/sbFormingControlActions/sbFrictionRegressorRS2/frictionRegressorFunctionRS2 ==
  data: v input; z input; Yf output; L input; Fd input; frictionRS2 parameter
function Yf = frictionRegressor(v,z,L, Fd, frictionRS2)

    % Forms the friction regressor from Zhu, W. H., & Piedboeuf, J. C. 
    % (2005). Adaptive output force tracking control of hydraulic cylinders 
    % with applications to robot manipulators.
    Yf = [(1 - L)*g(z, frictionRS2.zss)*S(z),...
          -(1 - L)*g(-z, frictionRS2.zss)*S(-z),...
          1 - L,...
          (1 - L)*S(v)*phivp(v)*v,...
          (1 - L)*S(-v)*phivn(v)*v,...
          S(Fd)*L*phifp(Fd,frictionRS2.deltap),...
          S(-Fd)*L*phifn(Fd,frictionRS2.deltan)];

end

function S = S(x)

    % Per (2) from Zhu, W. H., & Piedboeuf, J. C. (2005).
    if x > 0
        S = 1;
    else
        S = 0;
    end

end

function g = g(z, zss)

    % Per (5) in Zhu, W. H., & Piedboeuf, J. C. (2005).
    if z >= zss
        g = 1;
    elseif z <= 0
        g = 0;
    else
        g = z/zss;
    end

end

function phifp = phifp(f, deltafp)

    % Per (6) in Zhu, W. H., & Piedboeuf, J. C. (2005).
    phifp = f/(1 + deltafp*abs(f));

end

function phifn = phifn(f, deltafn)

    % Per (6) in Zhu, W. H., & Piedboeuf, J. C. (2005).
    phifn = f/(1 + deltafn*abs(f));

end

function phivp = phivp(v)

    % Chosen as constant. More details on pp. 211 of Zhu, W. H., & 
    % Piedboeuf, J. C. (2005), just above Eq. (71)
    phivp = 5 + 0*v;

end

function phivn = phivn(v)

    % Chosen as constant. More details on pp. 211 of Zhu, W. H., & 
    % Piedboeuf, J. C. (2005), just above Eq. (71)
    phivn = 5 + 0*v;

end

== matlab function VDCHyd2020a/sbVDCController/sbFormingControlActions/sbFrictionRegressorRS1/frictionRegressorFunctionRS1 ==
  data: v input; z input; Yf output; L input; Fd input; frictionRS1 parameter
function Yf = frictionRegressor(v,z,L, Fd, frictionRS1)

    % Forms the friction regressor from Zhu, W. H., & Piedboeuf, J. C. 
    % (2005). Adaptive output force tracking control of hydraulic cylinders 
    % with applications to robot manipulators.
    Yf = [(1 - L)*g(z, frictionRS1.zss)*S(z),...
          -(1 - L)*g(-z, frictionRS1.zss)*S(-z),...
          1 - L,...
          (1 - L)*S(v)*phivp(v)*v,...
          (1 - L)*S(-v)*phivn(v)*v,...
          S(Fd)*L*phifp(Fd,frictionRS1.deltap),...
          S(-Fd)*L*phifn(Fd,frictionRS1.deltan)];

end

function S = S(x)

    % Per (2) from Zhu, W. H., & Piedboeuf, J. C. (2005).
    if x > 0
        S = 1;
    else
        S = 0;
    end

end

function g = g(z, zss)

    % Per (5) in Zhu, W. H., & Piedboeuf, J. C. (2005).
    if z >= zss
        g = 1;
    elseif z <= 0
        g = 0;
    else
        g = z/zss;
    end

end

function phifp = phifp(f, deltafp)

    % Per (6) in Zhu, W. H., & Piedboeuf, J. C. (2005).
    phifp = f/(1 + deltafp*abs(f));

end

function phifn = phifn(f, deltafn)

    % Per (6) in Zhu, W. H., & Piedboeuf, J. C. (2005).
    phifn = f/(1 + deltafn*abs(f));

end

function phivp = phivp(v)

    % Chosen as constant. More details on pp. 211 of Zhu, W. H., & 
    % Piedboeuf, J. C. (2005), just above Eq. (71)
    phivp = 5 + 0*v;

end

function phivn = phivn(v)

    % Chosen as constant. More details on pp. 211 of Zhu, W. H., & 
    % Piedboeuf, J. C. (2005), just above Eq. (71)
    phivn = 5 + 0*v;

end

== matlab function VDCHyd2020a/sbHydraulicElements/sbValveFlowsRS1/liftValveFlows ==
  data: pa1 input; Qa1 output; pb1 input; u1v input; pS input; pR input; Qb1 output; valve1 parameter
function [Qa1, Qb1] = liftValveFlows(pa1, pb1, u1v, pS, pR, valve1)

    % Calculates lift valve flows per the paper equations (82) and (83).
    Qa1 = valve1.cp1*sqAbsPresDrop(pS - pa1)*u1v*selFcn(u1v) + ...
          valve1.cn1*sqAbsPresDrop(pa1 - pR)*u1v*selFcn(-u1v);
    Qb1 = -valve1.cn2*sqAbsPresDrop(pb1 - pR)*u1v*selFcn(u1v) - ...
          valve1.cp2*sqAbsPresDrop(pS - pb1)*u1v*selFcn(-u1v);
   
end

function S = selFcn(U)

    % Implements the selection function (84).
    if U > 0
        S = 1;
    else
        S = 0;
    end
    
end

function nup = sqAbsPresDrop(dp)

    % Implements the pressure drop function (85).
    nup = sign(dp)*sqrt(abs(dp));

end

== matlab function VDCHyd2020a/sbHydraulicElements/sbValveFlowsRS2/tiltValveFlows ==
  data: pa2 input; Qa2 output; pb2 input; u2v input; pS input; pR input; Qb2 output; valve2 parameter
function [Qa2, Qb2] = tiltValveFlows(pa2, pb2, u2v, pS, pR, valve2)

    % Calculates tilt valve flows per the paper equations (82) and (83).
    Qa2 = valve2.cp1*sqAbsPresDrop(pS - pa2)*u2v*selFcn(u2v) + ...
       valve2.cn1*sqAbsPresDrop(pa2 - pR)*u2v*selFcn(-u2v);
    Qb2 = -valve2.cn2*sqAbsPresDrop(pb2 - pR)*u2v*selFcn(u2v) - ...
       valve2.cp2*sqAbsPresDrop(pS - pb2)*u2v*selFcn(-u2v);
   
end

function S = selFcn(U)

    % Implements the selection function (84).    
    if U > 0
        S = 1;
    else
        S = 0;
    end
    
end

function nup = sqAbsPresDrop(dp)

    % Implements the pressure drop function (85).
    nup = sign(dp)*sqrt(abs(dp));

end

== matlab function VDCHyd2020a/sbVDCController/sbFormTotalRequiredForces/sbTotalRequiredForcesPS2/regressorYB52r ==
  data: B52Vr input; B52dVr input; B52V input; B52_Rot_W input; gravity parameter; YB52r output
function YB52r  = inertiaRegressor(B52Vr, B52dVr, B52V, B52_Rot_W,  gravity)

    % Forms regressor matrix YB42r as described in Appendix A of
    % Zhu, Wen-Hong. Virtual decomposition control: toward hyper degrees
    % of freedom robots. Vol. 60. Springer Science & Business Media, 2010.

    % The code below is not the most apparent 1-to-1 visual mapping to the
    % book equations since it was generated using a symbolic toolbox.

    vxr = B52Vr(1); vyr = B52Vr(2); vzr = B52Vr(3);
    wxr = B52Vr(4); wyr = B52Vr(5); wzr = B52Vr(6);
    
    axr = B52dVr(1); ayr = B52dVr(2); azr = B52dVr(3);
    dwxr = B52dVr(4); dwyr = B52dVr(5); dwzr = B52dVr(6);
    
    wx = B52V(4); wy = B52V(5); wz = B52V(6);
    
    B52g = B52_Rot_W*gravity.Wg;
    
    gx = B52g(1); gy = B52g(2); gz = B52g(3);
    
    Y11 = (-vyr * wz + vzr * wy + axr + gx);
    t5 = (wy * wyr);
    t6 = (wz * wzr);
    Y12 = -t5 - t6;
    t7 = (wxr * wy);
    Y13 = (t7 - dwzr);
    t8 = (wxr * wz);
    Y14  = (t8 + dwyr);
    Y15 = 0;
    Y16 = 0;
    Y17 = 0;
    Y18  = 0;
    Y19 = 0;
    Y110 = 0;
    Y111 = 0;
    Y112 = 0;
    Y113 = 0;
    Y21 = vxr * wz - vzr * wx + ayr + gy;
    t11 = wx * wyr;
    Y22 = t11 + dwzr;
    t12 = wx * wxr;
    Y23 = -t12 - t6;
    t13 = wyr * wz;
    Y24 = t13 - dwxr;
    Y25 = 0;
    Y26 = 0;
    Y27 = 0;
    Y28 = 0;
    Y29 = 0;
    Y210 = 0;
    Y211 = 0;
    Y212 = 0;
    Y213 = 0;
    Y31 = -vxr * wy + vyr * wx + azr + gz;
    t16 = wx * wzr;
    Y32 = t16 - dwyr;
    t17 = wy * wzr;
    Y33 = t17 + dwxr;
    Y34 = -t12 - t5;
    Y35 = 0;
    Y36 = 0;
    Y37 = 0;
    Y38 = 0;
    Y39 = 0;
    Y310 = 0;
    Y311 = 0;
    Y312 = 0;
    Y313 = 0;
    Y41 = 0;
    Y42 = 0;
    Y43 = Y31;
    Y44 = -Y21;
    Y45 = 0;
    Y46 = Y33;
    Y47 = -Y24;
    Y48 = Y32;
    Y49 = -Y22;
    Y410 = -t5 + t6;
    Y411 = t17 - t13 + dwxr;
    Y412 = -t13;
    Y413 = t17;
    Y51 = 0;
    Y52 = -Y43;
    Y53 = 0;
    Y54 = Y11;
    Y55 = -Y48;
    Y56 = 0;
    Y57 = Y14;
    Y58 = -Y46;
    Y59 = t12 - t6;
    Y510 = Y13;
    Y511 = t8;
    Y512 = -t16 + Y511 + dwyr;
    Y513 = -t16;
    Y61 = 0;
    Y62 = Y21;
    Y63 = -Y54;
    Y64 = 0;
    Y65 = Y22;
    Y66 = -Y510;
    Y67 = 0;
    Y68 = -t12 + t5;
    Y69 = Y24;
    Y610 = -Y57;
    Y611 = -t7;
    Y612 = t11;
    Y613 = Y612 + Y611 + dwzr;
    
    
    YB52r = [Y11 Y12 Y13 Y14 Y15 Y16 Y17 Y18 Y19 Y110 Y111 Y112 Y113;...
             Y21 Y22 Y23 Y24 Y25 Y26 Y27 Y28 Y29 Y210 Y211 Y212 Y213;...
             Y31 Y32 Y33 Y34 Y35 Y36 Y37 Y38 Y39 Y310 Y311 Y312 Y313;...
             Y41 Y42 Y43 Y44 Y45 Y46 Y47 Y48 Y49 Y410 Y411 Y412 Y413;...
             Y51 Y52 Y53 Y54 Y55 Y56 Y57 Y58 Y59 Y510 Y511 Y512 Y513;...
             Y61 Y62 Y63 Y64 Y65 Y66 Y67 Y68 Y69 Y610 Y611 Y612 Y613];

end

== matlab function VDCHyd2020a/sbVDCController/sbFormAnalyticQuantities/sbRevoluteSegment1/sbGeomPropRS1/sbLiftPistonVelocity/liftPistonVelocity ==
  data: dq1 input; x1 input; q1 input; dx1 output; geom parameter; cyl1 parameter
function dx1 = liftPistonVelocity(dq1, x1, q1, geom, cyl1)

    % Calculates lift piston velocity per the paper equation (21).
    dx1 = -(geom.L1*geom.L11*sin(q1))/(x1+cyl1.x0)*dq1;

end

== matlab function VDCHyd2020a/sbVDCController/sbFormAnalyticQuantities/sbRevoluteSegment1/sbGeomPropRS1/sbq11AngleVelocity/q11AngleRate ==
  data: x1 input; q11 input; dx1 input; dq11 output; geom parameter; cyl1 parameter
function dq11 = q11AngleRate(x1, q11, dx1, geom, cyl1)
    
    % Calculates q11 angle rate per the paper equation (22).
    dq11 = -((x1+cyl1.x0)-geom.L1*cos(q11))/((x1+cyl1.x0)*geom.L1*sin(q11))*dx1;

end

== matlab function VDCHyd2020a/sbVDCController/sbFormAnalyticQuantities/sbRevoluteSegment1/sbGeomPropRS1/sbq12AngleRate/q12AngleRate ==
  data: x1 input; q12 input; dx1 input; dq12 output; geom parameter; cyl1 parameter
function dq12 = q12AngleRate(x1, q12, dx1, geom, cyl1)

    % Calculates q12 angle rate per the paper equation (23). 
    dq12 = -((x1+cyl1.x0)-geom.L11*cos(q12))/((x1+cyl1.x0)*geom.L11*sin(q12))*dx1;

end

== matlab function VDCHyd2020a/sbVDCController/sbFormAnalyticQuantities/sbRevoluteSegment1/sbPosVecsRS1/B31_r_B31B41 ==
  data: x1 input; B31_r_B31B41 output; posVec parameter
function B31_r_B31B41 = B31_r_B31B41(x1, posVec)

    % position vector of {B41} frame at lift piston tip w.r.t. {B31} frame at 
    % lift cylinder connection point [m]
    B31_r_B31B41 = posVec.B31_r_B31B31p + [x1;0;0];

end

== matlab function VDCHyd2020a/sbVDCController/sbFormAnalyticQuantities/sbRevoluteSegment1/sbRotMatsRS1/B41_Rot_Tc1 ==
  data: q12 input; B41_Rot_Tc1 output
function B41_Rot_Tc1 = B41_Rot_Tc1(q12)

    B41_Rot_Tc1 = [+cos(q12) -sin(q12) 0;...
                   +sin(q12) +cos(q12) 0;...
                       0        0      1];

end

== matlab function VDCHyd2020a/sbVDCController/sbFormAnalyticQuantities/sbRevoluteSegment1/sbRotMatsRS1/Bc1_Rot_B11 ==
  data: q1 input; Bc1_Rot_B11 output
function Bc1_Rot_B11 = Bc1_Rot_B11(q1)

    Bc1_Rot_B11 = [+cos(q1) -sin(q1) 0;...
                   +sin(q1) +cos(q1) 0;...
                      0        0     1];

end
